simulink model "req8"  (R2019a)
settings: Solver=FixedStepAuto  StartTime=0.0  StopTime=100  RelTol=1e-3
settings Model: Creator=e40014285  LastModifiedBy=e40014285
settings ConfigComp: CovEnable=on  CovScope=ReferencedModels  RecordCoverage=on  DVModelCoverageObjectives=MCDC  DVTestSuiteOptimization=Auto  DVDetectOutOfBounds=on  DVRebuildModelRepresentation=Always

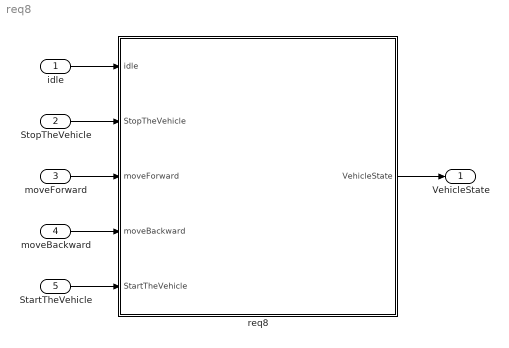
== system req8 ==
  idle : Inport
  StopTheVehicle : Inport  Port=2
  moveForward : Inport  Port=3
  moveBackward : Inport  Port=4
  StartTheVehicle : Inport  Port=5
  req8 : Stateflow chart  BlockKeywords=__PRM__SERIALIZED__DATA__:Stateflow Chart,Stateflow Diagram  TreatAsAtomicUnit=on
  VehicleState : Outport
  wires:
  moveBackward/1 -> req8/4(moveBackward)
  StartTheVehicle/1 -> req8/5(StartTheVehicle)
  idle/1 -> req8/1(idle)
  req8/1(VehicleState) -> VehicleState/1
  StopTheVehicle/1 -> req8/2(StopTheVehicle)
  moveForward/1 -> req8/3(moveForward)

== stateflow chart req8/req8 ==
  state OffState
    VehicleState=0;
  state VehicelStart
    state Idle
      VehicleState=1;
    state MoveForwad
      VehicleState=2;
    state MoveBackward
      VehicleState=3;
    (default) -> Idle
    MoveForwad -> Idle [order 1] : [idle]
    Idle -> MoveForwad [order 2] : [moveForward]
    MoveBackward -> Idle [order 1] : [idle]
    Idle -> MoveBackward [order 3] : [moveBackward]
    MoveBackward -> MoveForwad [order 2] : [moveForward]
    MoveForwad -> MoveBackward [order 2] : [moveBackward]
  (default) -> OffState
  OffState -> VehicelStart : [StartTheVehicle]
  Idle -> OffState [order 1] : [StopTheVehicle]
  data: idle input; StopTheVehicle input; moveForward input; moveBackward input; StartTheVehicle input; VehicleState output
